simulink model "dxqq08022311"  (R2022b)
settings: Solver=ode45  StartTime=0.0  StopTime=0.24  MaxStep=0.0001  RelTol=1e-4
libraries: spsThyristorLib x4, spsVoltageMeasurementLib x4, spsACVoltageSourceLib x2, spsGroundLib x2, spsLinearTransformerLib x2, spsSeriesRLCBranchLib x2, spsCurrentMeasurementLib x1, spsUniversalBridgeLib x1, spspowerguiLib x1
settings Model: Creator=Zachary  LastModifiedBy=ASUS
settings DebuggingCC: UnconnectedInputMsg=warning  UnconnectedOutputMsg=warning  UnconnectedLineMsg=warning
settings ModelReferenceCC: EnableRefExpFcnMdlSchedulingChecks=on
settings RTWCC: DLArmComputeVersion=19.05

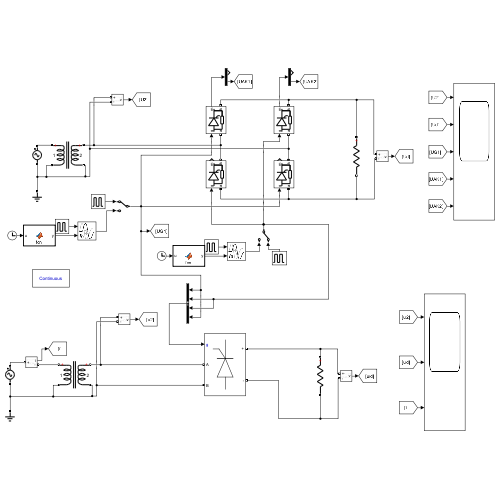
[thumbnail: Simulink's stored preview of the top-level diagram]
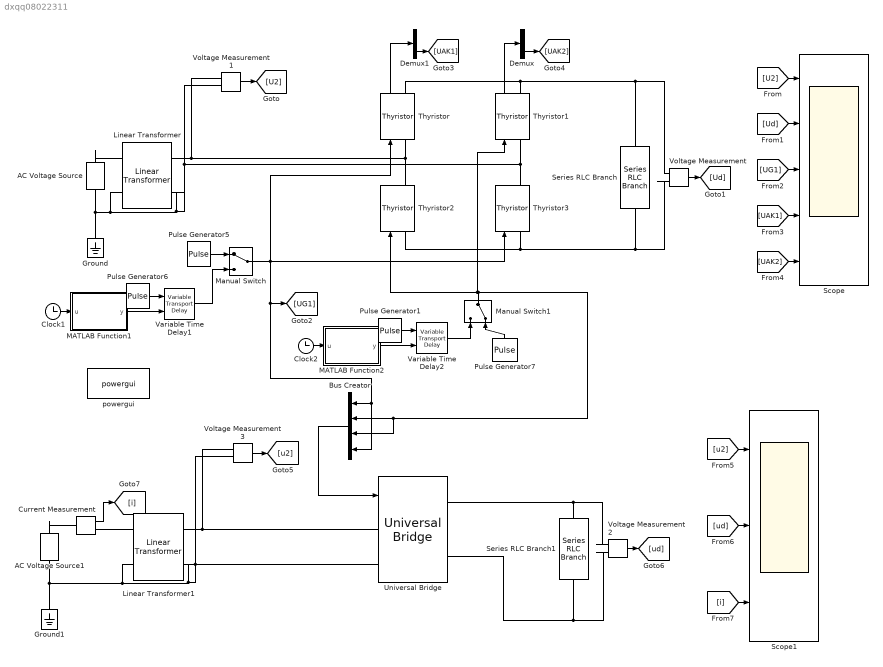
== system dxqq08022311 ==
  AC Voltage Source : spsACVoltageSourceLib/AC Voltage Source  Amplitude=100*sqrt(2)  Phase=0  Frequency=50  SampleTime=0  Measurements=None  BusType=swing  Pref=10e3  Qref=0  Qmin=-inf  Qmax=+inf
  AC Voltage Source1 : spsACVoltageSourceLib/AC Voltage Source  Amplitude=100*sqrt(2)  Phase=0  Frequency=50  SampleTime=0  Measurements=None  BusType=swing  Pref=10e3  Qref=0  Qmin=-inf  Qmax=+inf
  Bus Creator : BusCreator  Inputs=4
  Clock1 : Clock
  Clock2 : Clock
  Current Measurement : spsCurrentMeasurementLib/Current Measurement  PhasorSimulation=off  OutputType=Complex  PSBequivalent=0
  Demux : Demux  Outputs=2
  Demux1 : Demux  Outputs=2
  Ground : spsGroundLib/Ground  LConnTagsString=a
  Ground1 : spsGroundLib/Ground  LConnTagsString=a
  Linear Transformer : spsLinearTransformerLib/Linear Transformer  UNITS=pu  NominalPower=[250e6 50 ]  winding1=[735e3 0 0]  winding2=[315e3 0 0]  ThreeWindings=off  winding3=[ 315e3 0.002 0.08 ]  RmLm=[ 500 500 ]  Measurements=None  DataType=off
  Linear Transformer1 : spsLinearTransformerLib/Linear Transformer  UNITS=pu  NominalPower=[250e6 50 ]  winding1=[735e3 0 0]  winding2=[315e3 0 0]  ThreeWindings=off  winding3=[ 315e3 0.002 0.08 ]  RmLm=[ 500 500 ]  Measurements=None  DataType=off
  MATLAB Function1 : MATLAB Function  TreatAsAtomicUnit=on
  MATLAB Function2 : MATLAB Function  TreatAsAtomicUnit=on
  Manual Switch : ManualSwitch
  Manual Switch1 : ManualSwitch  CurrentSetting=0
  Pulse Generator1 : DiscretePulseGenerator  PulseType=Time based  Amplitude=50  Period=0.02  PulseWidth=5  PhaseDelay=180*0.02/360
  Pulse Generator5 : DiscretePulseGenerator  PulseType=Time based  Amplitude=50  Period=0.02  PulseWidth=5  PhaseDelay=30*0.02/360
  Pulse Generator6 : DiscretePulseGenerator  PulseType=Time based  Amplitude=50  Period=0.02  PulseWidth=5  PhaseDelay=0*0.02/360
  Pulse Generator7 : DiscretePulseGenerator  PulseType=Time based  Amplitude=50  Period=0.02  PulseWidth=5  PhaseDelay=210*0.02/360
  Scope : Scope  NumInputPorts=5
  Scope1 : Scope  NumInputPorts=3
  Series RLC Branch : spsSeriesRLCBranchLib/Series RLC Branch  LConnTagsString=__new0  RConnTagsString=__new0  BranchType=R  Resistance=10  Inductance=1e-3  SetiL0=off  InitialCurrent=0  Capacitance=1e-6  Setx0=off  InitialVoltage=0  Measurements=None
  Series RLC Branch1 : spsSeriesRLCBranchLib/Series RLC Branch  LConnTagsString=__new0  RConnTagsString=__new0  BranchType=R  Resistance=10  Inductance=1e-3  SetiL0=off  InitialCurrent=0  Capacitance=1e-6  Setx0=off  InitialVoltage=0  Measurements=None
  Thyristor{,1..3} (4 alike) : spsThyristorLib/Thyristor  Ron=0.00001  Lon=0  Vf=0  IC=0  Rs=500  Cs=250e-9  Measurements=on
  Universal Bridge : spsUniversalBridgeLib/Universal Bridge  Arms=2  SnubberResistance=1e5  SnubberCapacitance=inf  Device=Thyristors  Ron=1e-3  Lon=0  ForwardVoltages="[  0  0  ]"  ForwardVoltage=0  GTOparameters=[ 10e-6 , 20e-6 ]  IGBTparameters=[ 1e-6 , 2e-6 ]  Measurements=None  Measurements_2=None  converterType=Rectifier
  Variable Time Delay1 : VariableTransportDelay  MaximumDelay=360*0.02/360  InitialOutput=0*0.02/360
  Variable Time Delay2 : VariableTransportDelay  MaximumDelay=360*0.02/360  InitialOutput=180*0.02/360
  Voltage Measurement{,1..3} (4 alike) : spsVoltageMeasurementLib/Voltage Measurement  PhasorSimulation=off  OutputType=Complex  PSBequivalent=0
  powergui : spspowerguiLib/powergui  Priority=1  SimulationMode=Continuous  SampleTime=50e-6  frequency=60  Iterations=50  frequencyindice=50  Pbase=100e6  ErrMax=1e-4  UnitsV=kV  UnitsW=MW  buscounter=0  FunctionMessages=off  echomessages=off  EnableUseOfTLC=off  CurrentSourceSwitches=off  DisableSnubberDevices=off  DisableRonSwitches=off  DisableVfSwitches=off  DisplayEquations=off  AutomaticDiscreteSolvers=off  SolverType=Tustin/Backward Euler (TBE)  Interpol=off  ExternalGateDelay=off  methode=off  Ts=100  x0status=blocks  SPID=on  SwTol=0  HookPort=off  NonlinearTolerance=1e-4  nMaxIteration=100  ContinueOnMaxIteration=off  RestoreLinks=warning  ResistiveCurrentMeasurement=off  Frange=[0:2:500]  Ylog=off  Xlog=on  ShowGrid=off  save=off  variable=ZData  structure=0  ZoomFFT=off  StartTime=0.0  cycles=1  DisplayStyle=1  fundamental=60  FreqAxis=off  MaxFrequency=1000  frequencyindicesteady=1  RmsSteady=1  display=off
  wires:
  [U2] -> Scope/1
  Voltage Measurement1/1 -> [U2]
  Voltage Measurement/1 -> [Ud]
  [Ud] -> Scope/2
  Variable Time Delay1/1 -> Manual Switch/2
  [UG1] -> Scope/3
  Thyristor1/1 -> Demux/1
  Thyristor/1 -> Demux1/1
  Demux1/2 -> [UAK1]
  Demux/2 -> [UAK2]
  [UAK2] -> Scope/5
  [UAK1] -> Scope/4
  [i] -> Scope1/3
  Voltage Measurement2/1 -> [ud]
  Voltage Measurement3/1 -> [u2]
  [u2] -> Scope1/1
  Current Measurement/1 -> [i]
  [ud] -> Scope1/2
  Bus Creator/1 -> Universal Bridge/1
  Manual Switch/1 -> Thyristor3/1, Thyristor/1, Bus Creator/4, Bus Creator/1, [UG1]
  Manual Switch1/1 -> Bus Creator/3, Bus Creator/2, Thyristor2/1, Thyristor1/1
  Pulse Generator6/1 -> Variable Time Delay1/1
  Clock1/1 -> MATLAB Function1/1(u)
  MATLAB Function1/1(y) -> Variable Time Delay1/2
  MATLAB Function2/1(y) -> Variable Time Delay2/2
  Pulse Generator1/1 -> Variable Time Delay2/1
  Clock2/1 -> MATLAB Function2/1(u)
  Pulse Generator5/1 -> Manual Switch/1
  Variable Time Delay2/1 -> Manual Switch1/1
  Pulse Generator7/1 -> Manual Switch1/2
  connections:
  Thyristor/LConn1 -- Voltage Measurement1/LConn1 -- Linear Transformer/RConn1 -- Thyristor2/RConn1
  Thyristor1/LConn1 -- Linear Transformer/LConn2 -- Ground/LConn1 -- AC Voltage Source/LConn1 -- Linear Transformer/RConn2 -- Voltage Measurement1/LConn2 -- Thyristor3/RConn1
  Series RLC Branch/LConn1 -- Thyristor/RConn1 -- Thyristor1/RConn1 -- Voltage Measurement/LConn1
  Thyristor2/LConn1 -- Series RLC Branch/RConn1 -- Voltage Measurement/LConn2 -- Thyristor3/LConn1
  AC Voltage Source/RConn1 -- Linear Transformer/LConn1
  Linear Transformer1/RConn2 -- Universal Bridge/LConn2 -- Voltage Measurement3/LConn2 -- Linear Transformer1/LConn2 -- Ground1/LConn1 -- AC Voltage Source1/LConn1
  Universal Bridge/RConn2 -- Voltage Measurement2/LConn2 -- Series RLC Branch1/RConn1
  Linear Transformer1/RConn1 -- Universal Bridge/LConn1 -- Voltage Measurement3/LConn1
  Voltage Measurement2/LConn1 -- Series RLC Branch1/LConn1 -- Universal Bridge/RConn1
  AC Voltage Source1/RConn1 -- Current Measurement/LConn1
  Current Measurement/RConn1 -- Linear Transformer1/LConn1

== matlab function dxqq08022311/MATLAB Function2 ==
  data: u input; y output
function y = fcn(u)

y = u*30/360;

== matlab function dxqq08022311/MATLAB Function1 ==
  data: u input; y output
function y = fcn(u)

y = u*30/360;
